simulink model "IM_model_final_2"  (R2021a)
settings: Solver=FixedStepAuto  StartTime=0.0  StopTime=10  FixedStep=1e-5  RelTol=1e-3
InitFcn:
  | %% Values of Parameters
  | R1a=0.001579662;
  | R2a=0.001130053590568;
  | X1a=0.0253956;
  | X2a=0.024186280814577;
  | Xma=0.744789315664148;
  | Rca=45.967698519515480;
  | 
  | %% Other Parameters
  | Power=4300e3;
  | Torque=34500;
  | pole=6;
  | pp=pole/2;
  | Vll=700;
  | f=60;
  | Jm=242.28;
  | 
  | 
  | %% Inductances
  | L1a=X1a/2/pi/f;
  | L2a=X2a/2/pi/f;
  | Lma=Xma/2/pi/f;
libraries: spsSeriesRLCBranchLib x6, spsACVoltageSourceLib x3, spsAsynchronousMachineSIUnitsLib x2, spsMeanLib x2, spsGroundLib x1, spspowerguiLib x1
settings Model: Creator=enes_  LastModifiedBy=enes_

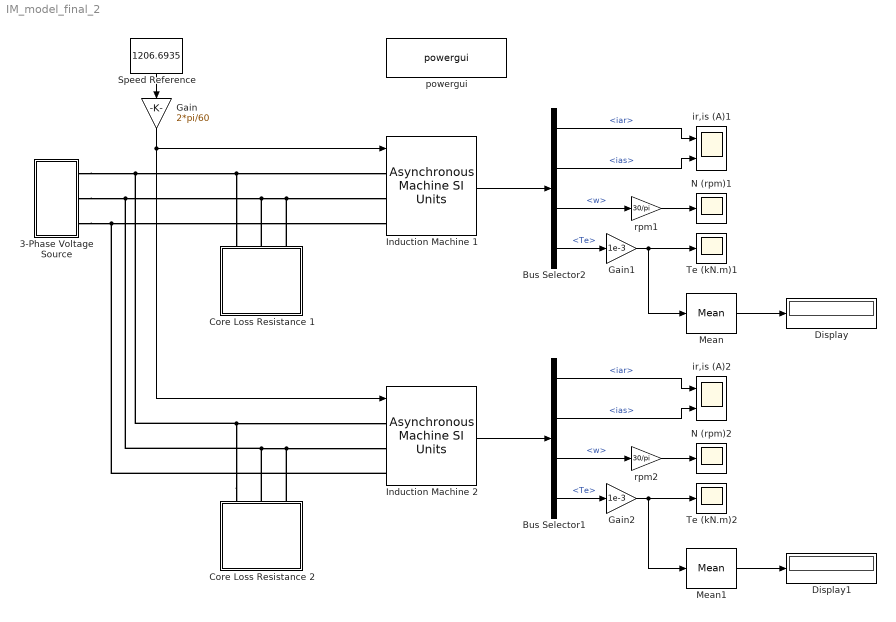
== system IM_model_final_2 ==
  3-Phase Voltage Source : Subsystem
  Bus Selector1 : BusSelector  OutputSignals=iar,ias,w,Te
  Bus Selector2 : BusSelector  OutputSignals=iar,ias,w,Te
  "Core Loss Resistance 1 " : Subsystem
  Core Loss Resistance 2 : Subsystem
  Display : Display
  Display1 : Display
  Gain : Gain  Gain=2*pi/60
  Gain1 : Gain  Gain=1e-3
  Gain2 : Gain  Gain=1e-3
  Induction Machine 1 : spsAsynchronousMachineSIUnitsLib/Asynchronous Machine SI Units  RotorType=Squirrel-cage  PresetModel=No  MechanicalLoad=Speed w  ShowDetailedParameters=on  ReferenceFrame=Stationary  Units=SI  MeasurementBus=on  NominalParameters=[Power/2 Vll f]  VoltageRatio=1  Stator=[R1a L1a]  Rotor=[R2a L2a]  Cage1=[ 0.022 0.226/377]  Cage2=[ 0.022 0.226/377]  Lm=Lma  Mechanical=[Jm 0 pp]  PolePairs=pp  InitialConditions="[ 1,0   0,0,0   0,0,0 ]"  SimulateSaturation=off  Saturation=[14.03593122, 27.81365428, 53.79336849, 72.68890987, 97.98006896, 148.6815601, 215.7428561, 302.9841135, 428.7778367 ; 230, 322, 414, 460, 506, 552, 598, 644, 690]  LoadFlowParameters=0  TsPowergui=0  TsBlock=-1  IterativeModel=Trapezoidal non iterative  IterativeDiscreteModel=Trapezoidal non iterative  Pmec=0
      settings: AttributesFormatString=\n
  Induction Machine 2 : spsAsynchronousMachineSIUnitsLib/Asynchronous Machine SI Units  RotorType=Squirrel-cage  PresetModel=No  MechanicalLoad=Speed w  ShowDetailedParameters=on  ReferenceFrame=Stationary  Units=SI  MeasurementBus=on  NominalParameters=[Power/2 Vll f]  VoltageRatio=1  Stator=[R1a L1a]  Rotor=[R2a L2a]  Cage1=[ 0.022 0.226/377]  Cage2=[ 0.022 0.226/377]  Lm=Lma  Mechanical=[Jm 0 pp]  PolePairs=pp  InitialConditions="[ 1,0   0,0,0   0,0,0 ]"  SimulateSaturation=off  Saturation=[14.03593122, 27.81365428, 53.79336849, 72.68890987, 97.98006896, 148.6815601, 215.7428561, 302.9841135, 428.7778367 ; 230, 322, 414, 460, 506, 552, 598, 644, 690]  LoadFlowParameters=0  TsPowergui=0  TsBlock=-1  IterativeModel=Trapezoidal non iterative  IterativeDiscreteModel=Trapezoidal non iterative  Pmec=0
      settings: AttributesFormatString=\n
  Mean : spsMeanLib/Mean  Freq=60  Vinit=0  Ts=0
  Mean1 : spsMeanLib/Mean  Freq=60  Vinit=0  Ts=0
  N (rpm)1 : Scope
  N (rpm)2 : Scope
  Speed Reference : Constant  Value=1206.6935
  Te (kN.m)1 : Scope
  Te (kN.m)2 : Scope
  ir,is (A)1 : Scope  NumInputPorts=2
  ir,is (A)2 : Scope  NumInputPorts=2
  powergui : spspowerguiLib/powergui  SimulationMode=Continuous  SampleTime=0  frequency=60  Iterations=50  frequencyindice=60  Pbase=100e6  ErrMax=1e-4  UnitsV=kV  UnitsW=MW  buscounter=0  FunctionMessages=off  echomessages=off  EnableUseOfTLC=off  CurrentSourceSwitches=off  DisableSnubberDevices=off  DisableRonSwitches=off  DisableVfSwitches=off  DisplayEquations=off  AutomaticDiscreteSolvers=off  SolverType=Tustin  Interpol=off  ExternalGateDelay=off  methode=off  Ts=0  x0status=blocks  SPID=on  SwTol=0  HookPort=off  NonlinearTolerance=1e-4  nMaxIteration=100  ContinueOnMaxIteration=off  RestoreLinks=warning  ResistiveCurrentMeasurement=off  Frange=[0:2:500]  Ylog=off  Xlog=on  ShowGrid=off  save=off  variable=ZData  structure=0  ZoomFFT=on  StartTime=0.0  cycles=1  DisplayStyle=1  fundamental=60  FreqAxis=off  MaxFrequency=1000  frequencyindicesteady=1  RmsSteady=1  display=off
  rpm1 : Gain  Gain=30/pi  SaturateOnIntegerOverflow=on  OutDataTypeStr=Inherit: Same as input  ParamDataTypeStr=Inherit: Same as input
  rpm2 : Gain  Gain=30/pi  SaturateOnIntegerOverflow=on  OutDataTypeStr=Inherit: Same as input  ParamDataTypeStr=Inherit: Same as input
  wires:
  Gain1/1 -> Mean/1, Te (kN.m)1/1
  Bus Selector2/2 -> ir,is (A)1/2  "<ias>"
  rpm1/1 -> N (rpm)1/1
  Bus Selector2/1 -> ir,is (A)1/1  "<iar>"
  Bus Selector2/4 -> Gain1/1  "<Te>"
  Induction Machine 1/1 -> Bus Selector2/1
  Bus Selector2/3 -> rpm1/1  "<w>"
  Speed Reference/1 -> Gain/1
  Mean/1 -> Display/1
  Gain/1 -> Induction Machine 1/1, Induction Machine 2/1
  Mean1/1 -> Display1/1
  Gain2/1 -> Mean1/1, Te (kN.m)2/1
  Induction Machine 2/1 -> Bus Selector1/1
  Bus Selector1/2 -> ir,is (A)2/2  "<ias>"
  Bus Selector1/1 -> ir,is (A)2/1  "<iar>"
  Bus Selector1/3 -> rpm2/1  "<w>"
  rpm2/1 -> N (rpm)2/1
  Bus Selector1/4 -> Gain2/1  "<Te>"
  connections:
  Core Loss Resistance 2/LConn2 -- Induction Machine 2/LConn2 -- Core Loss Resistance 2/LConn3 -- Induction Machine 1/LConn2 -- "Core Loss Resistance 1 "/LConn3 -- "Core Loss Resistance 1 "/LConn2 -- 3-Phase Voltage Source/RConn2
  3-Phase Voltage Source/RConn3 -- Induction Machine 1/LConn3 -- Induction Machine 2/LConn3
  Core Loss Resistance 2/LConn1 -- Induction Machine 2/LConn1 -- Induction Machine 1/LConn1 -- "Core Loss Resistance 1 "/LConn1 -- 3-Phase Voltage Source/RConn1

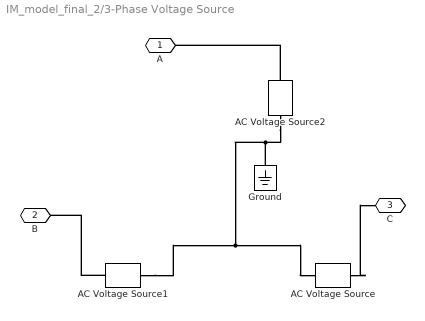
== system IM_model_final_2/3-Phase Voltage Source ==
  AC Voltage Source : spsACVoltageSourceLib/AC Voltage Source  Amplitude=Vll/sqrt(3)*sqrt(2)  Phase=120  Frequency=f  SampleTime=0  Measurements=None  BusType=swing  Pref=10e3  Qref=0  Qmin=-inf  Qmax=+inf
  AC Voltage Source1 : spsACVoltageSourceLib/AC Voltage Source  Amplitude=Vll/sqrt(3)*sqrt(2)  Phase=240  Frequency=f  SampleTime=0  Measurements=None  BusType=swing  Pref=10e3  Qref=0  Qmin=-inf  Qmax=+inf
  AC Voltage Source2 : spsACVoltageSourceLib/AC Voltage Source  Amplitude=Vll/sqrt(3)*sqrt(2)  Phase=0  Frequency=f  SampleTime=0  Measurements=None  BusType=swing  Pref=10e3  Qref=0  Qmin=-inf  Qmax=+inf
  Ground : spsGroundLib/Ground  LConnTagsString=a
  A : PMIOPort  Side=Right
  B : PMIOPort  Port=2  Side=Right
  C : PMIOPort  Port=3  Side=Right
  connections:
  AC Voltage Source2/LConn1 -- AC Voltage Source1/LConn1 -- AC Voltage Source/LConn1 -- Ground/LConn1
  AC Voltage Source1/RConn1 -- B/RConn1
  AC Voltage Source2/RConn1 -- A/RConn1
  AC Voltage Source/RConn1 -- C/RConn1

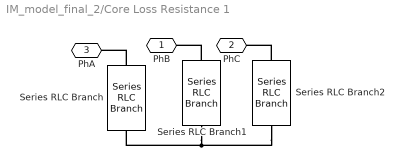
== system IM_model_final_2/Core Loss Resistance 1  ==
  Series RLC Branch : spsSeriesRLCBranchLib/Series RLC Branch  LConnTagsString=__new0  RConnTagsString=__new0  BranchType=R  Resistance=Rca  Inductance=1e-3  SetiL0=off  InitialCurrent=0  Capacitance=1e-6  Setx0=off  InitialVoltage=0  Measurements=None
  Series RLC Branch1 : spsSeriesRLCBranchLib/Series RLC Branch  LConnTagsString=__new0  RConnTagsString=__new0  BranchType=R  Resistance=Rca  Inductance=1e-3  SetiL0=off  InitialCurrent=0  Capacitance=1e-6  Setx0=off  InitialVoltage=0  Measurements=None
  Series RLC Branch2 : spsSeriesRLCBranchLib/Series RLC Branch  LConnTagsString=__new0  RConnTagsString=__new0  BranchType=R  Resistance=Rca  Inductance=1e-3  SetiL0=off  InitialCurrent=0  Capacitance=1e-6  Setx0=off  InitialVoltage=0  Measurements=None
  PhB : PMIOPort  Side=Left
  PhC : PMIOPort  Port=2  Side=Left
  PhA : PMIOPort  Port=3  Side=Left
  connections:
  Series RLC Branch2/RConn1 -- Series RLC Branch1/RConn1 -- Series RLC Branch/RConn1
  Series RLC Branch/LConn1 -- PhA/RConn1
  Series RLC Branch1/LConn1 -- PhB/RConn1
  Series RLC Branch2/LConn1 -- PhC/RConn1

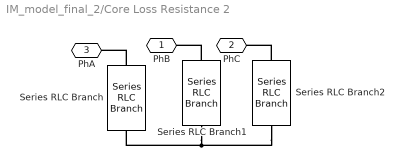
== system IM_model_final_2/Core Loss Resistance 2 ==
  Series RLC Branch : spsSeriesRLCBranchLib/Series RLC Branch  LConnTagsString=__new0  RConnTagsString=__new0  BranchType=R  Resistance=Rca  Inductance=1e-3  SetiL0=off  InitialCurrent=0  Capacitance=1e-6  Setx0=off  InitialVoltage=0  Measurements=None
  Series RLC Branch1 : spsSeriesRLCBranchLib/Series RLC Branch  LConnTagsString=__new0  RConnTagsString=__new0  BranchType=R  Resistance=Rca  Inductance=1e-3  SetiL0=off  InitialCurrent=0  Capacitance=1e-6  Setx0=off  InitialVoltage=0  Measurements=None
  Series RLC Branch2 : spsSeriesRLCBranchLib/Series RLC Branch  LConnTagsString=__new0  RConnTagsString=__new0  BranchType=R  Resistance=Rca  Inductance=1e-3  SetiL0=off  InitialCurrent=0  Capacitance=1e-6  Setx0=off  InitialVoltage=0  Measurements=None
  PhB : PMIOPort  Side=Left
  PhC : PMIOPort  Port=2  Side=Left
  PhA : PMIOPort  Port=3  Side=Left
  connections:
  Series RLC Branch2/RConn1 -- Series RLC Branch1/RConn1 -- Series RLC Branch/RConn1
  Series RLC Branch/LConn1 -- PhA/RConn1
  Series RLC Branch1/LConn1 -- PhB/RConn1
  Series RLC Branch2/LConn1 -- PhC/RConn1
